simulink model "FCS_Design"  (R2024b)
settings: Solver=FixedStepDiscrete  StartTime=0.0  StopTime=10.0  RelTol=1e-3
settings OptimizationCC: DefaultParameterBehavior=Inlined  EnhancedBackFolding=on  PassReuseOutputArgsAs=Individual arguments  ZeroExternalMemoryAtStartup=off  ZeroInternalMemoryAtStartup=off  OptimizeBlockOrder=speed  DifferentSizesBufferReuse=on  OptimizationCustomize=off  EfficientTunableParamExpr=on
settings DebuggingCC: ParameterTunabilityLossMsg=error
settings SFSimCC: MATLABDynamicMemAlloc=off
settings RTWCC: Description=Embedded Coder  SystemTargetFile=ert.tlc  TemplateMakefile=ert_default_tmf
settings CodeAppCC: ForceParamTrailComments=on  IgnoreCustomStorageClasses=off  OperatorAnnotations=on  SimulinkDataObjDesc=on  SFDataObjDesc=on  InsertBlockDesc=on
settings ERTTargetCC: TargetLangStandard=C99 (ISO)  GenerateSampleERTMain=on  ERTCustomFileTemplate=example_file_process.tlc

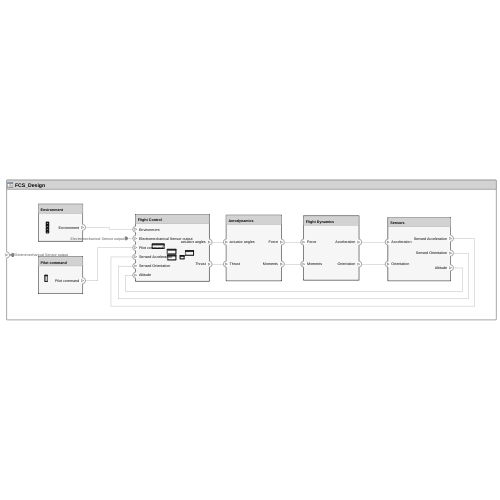
[thumbnail: Simulink's stored preview of the top-level diagram]
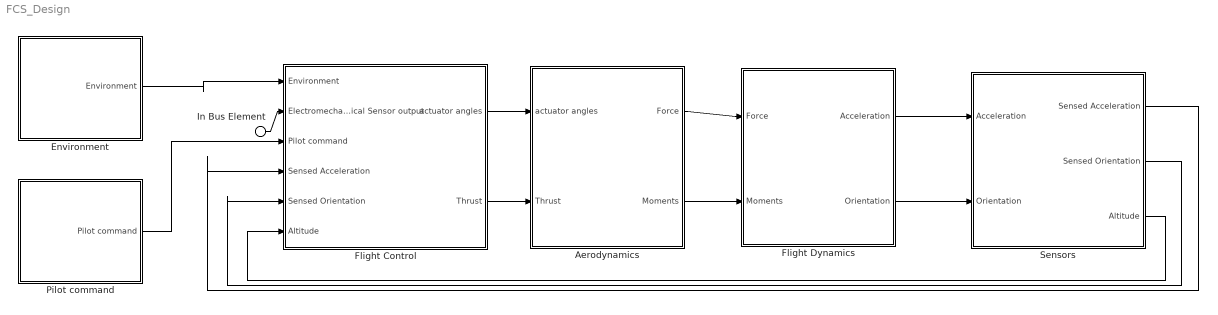
== system FCS_Design ==
  In Bus Element : Inport  PortName=Electromechanical Sensor output
  Aerodynamics : Subsystem
      settings: PortSchema="{\"entries\":[{\"content\":{\"headerSize\":26,\"margin\":15,\"minimumSpacing\":25,\"sides\":[{\"content\":{\"connectorIds\":[\"In1\",\"In2\"]},\"type\":\"ConnectorPlacement.EquallySpacedRectSide\",\"uuid\":\"d5d2077c-3b21-4d02-aba8-81a870ce330d\"},{\"content\":{\"connectorIds\":[\"Out1\",\"Out2\"],\"side\":\"RIGHT\"},\"type\":\"ConnectorPlacement.EquallySpacedRectSide\",\"uuid\":\"4fd2a41b-7df5-4294-829e-ab8ed7c0ae08\"},{\"content\":{\"side\":\"TOP\"},\"type\":\"ConnectorPlacement.EquallySpacedRectSide\",\"uuid\":\"02481d6b-9835-4bb6-a897-737025ba9b9d\"}]},\"type\":\"ConnectorPlacement.EquallySpacedConnector\",\"uuid\":\"7e1f026a-fb6c-4dac-9805-315e8c94a54c\"}],\"packageUris\":[\"http://schema.mathworks.com/mf0/Connector/R2020b\"],\"version\":\"1.0\"}"
  Environment : Subsystem
      settings: PortSchema="{\"entries\":[{\"content\":{\"headerSize\":26,\"margin\":15,\"minimumSpacing\":25,\"sides\":[{\"content\":{},\"type\":\"ConnectorPlacement.EquallySpacedRectSide\",\"uuid\":\"d5d2077c-3b21-4d02-aba8-81a870ce330d\"},{\"content\":{\"connectorIds\":[\"Out1\"],\"side\":\"RIGHT\"},\"type\":\"ConnectorPlacement.EquallySpacedRectSide\",\"uuid\":\"4fd2a41b-7df5-4294-829e-ab8ed7c0ae08\"},{\"content\":{\"side\":\"TOP\"},\"type\":\"ConnectorPlacement.EquallySpacedRectSide\",\"uuid\":\"02481d6b-9835-4bb6-a897-737025ba9b9d\"}]},\"type\":\"ConnectorPlacement.EquallySpacedConnector\",\"uuid\":\"7e1f026a-fb6c-4dac-9805-315e8c94a54c\"}],\"packageUris\":[\"http://schema.mathworks.com/mf0/Connector/R2020b\"],\"version\":\"1.0\"}"
  Flight Control : Subsystem
      settings: PortSchema="{\"entries\":[{\"content\":{\"headerSize\":26,\"margin\":15,\"minimumSpacing\":25,\"sides\":[{\"content\":{\"connectorIds\":[\"In1\",\"In2\",\"In3\",\"In4\",\"In5\",\"In6\"]},\"type\":\"ConnectorPlacement.EquallySpacedRectSide\",\"uuid\":\"d5d2077c-3b21-4d02-aba8-81a870ce330d\"},{\"content\":{\"connectorIds\":[\"Out1\",\"Out2\"],\"side\":\"RIGHT\"},\"type\":\"ConnectorPlacement.EquallySpacedRectSide\",\"uuid\":\"4fd2a41b-7df5-4294-829e-ab8ed7c0ae08\"},{\"content\":{\"side\":\"TOP\"},\"type\":\"ConnectorPlacement.EquallySpacedRectSide\",\"uuid\":\"02481d6b-9835-4bb6-a897-737025ba9b9d\"}]},\"type\":\"ConnectorPlacement.EquallySpacedConnector\",\"uuid\":\"7e1f026a-fb6c-4dac-9805-315e8c94a54c\"}],\"packageUris\":[\"http://schema.mathworks.com/mf0/Connector/R2020b\"],\"version\":\"1.0\"}"
  Flight Dynamics : Subsystem
      settings: PortSchema="{\"entries\":[{\"content\":{\"headerSize\":26,\"margin\":15,\"minimumSpacing\":25,\"sides\":[{\"content\":{\"connectorIds\":[\"In1\",\"In2\"]},\"type\":\"ConnectorPlacement.EquallySpacedRectSide\",\"uuid\":\"d5d2077c-3b21-4d02-aba8-81a870ce330d\"},{\"content\":{\"connectorIds\":[\"Out1\",\"Out2\"],\"side\":\"RIGHT\"},\"type\":\"ConnectorPlacement.EquallySpacedRectSide\",\"uuid\":\"4fd2a41b-7df5-4294-829e-ab8ed7c0ae08\"},{\"content\":{\"side\":\"TOP\"},\"type\":\"ConnectorPlacement.EquallySpacedRectSide\",\"uuid\":\"02481d6b-9835-4bb6-a897-737025ba9b9d\"}]},\"type\":\"ConnectorPlacement.EquallySpacedConnector\",\"uuid\":\"7e1f026a-fb6c-4dac-9805-315e8c94a54c\"}],\"packageUris\":[\"http://schema.mathworks.com/mf0/Connector/R2020b\"],\"version\":\"1.0\"}"
  Pilot command : Subsystem
      settings: PortSchema="{\"entries\":[{\"content\":{\"headerSize\":26,\"margin\":15,\"minimumSpacing\":25,\"sides\":[{\"content\":{},\"type\":\"ConnectorPlacement.EquallySpacedRectSide\",\"uuid\":\"d5d2077c-3b21-4d02-aba8-81a870ce330d\"},{\"content\":{\"connectorIds\":[\"Out1\"],\"side\":\"RIGHT\"},\"type\":\"ConnectorPlacement.EquallySpacedRectSide\",\"uuid\":\"4fd2a41b-7df5-4294-829e-ab8ed7c0ae08\"},{\"content\":{\"side\":\"TOP\"},\"type\":\"ConnectorPlacement.EquallySpacedRectSide\",\"uuid\":\"02481d6b-9835-4bb6-a897-737025ba9b9d\"}]},\"type\":\"ConnectorPlacement.EquallySpacedConnector\",\"uuid\":\"7e1f026a-fb6c-4dac-9805-315e8c94a54c\"}],\"packageUris\":[\"http://schema.mathworks.com/mf0/Connector/R2020b\"],\"version\":\"1.0\"}"
  Sensors : Subsystem
      settings: PortSchema="{\"entries\":[{\"content\":{\"headerSize\":26,\"margin\":15,\"minimumSpacing\":25,\"sides\":[{\"content\":{\"connectorIds\":[\"In1\",\"In2\"]},\"type\":\"ConnectorPlacement.EquallySpacedRectSide\",\"uuid\":\"d5d2077c-3b21-4d02-aba8-81a870ce330d\"},{\"content\":{\"connectorIds\":[\"Out1\",\"Out2\",\"Out3\"],\"side\":\"RIGHT\"},\"type\":\"ConnectorPlacement.EquallySpacedRectSide\",\"uuid\":\"4fd2a41b-7df5-4294-829e-ab8ed7c0ae08\"},{\"content\":{\"side\":\"TOP\"},\"type\":\"ConnectorPlacement.EquallySpacedRectSide\",\"uuid\":\"02481d6b-9835-4bb6-a897-737025ba9b9d\"}]},\"type\":\"ConnectorPlacement.EquallySpacedConnector\",\"uuid\":\"7e1f026a-fb6c-4dac-9805-315e8c94a54c\"}],\"packageUris\":[\"http://schema.mathworks.com/mf0/Connector/R2020b\"],\"version\":\"1.0\"}"
  wires:
  Flight Dynamics/1(Acceleration) -> Sensors/1(Acceleration)
  Flight Dynamics/2(Orientation) -> Sensors/2(Orientation)
  Sensors/3(Altitude) -> Flight Control/6(Altitude)
  Sensors/2(Sensed Orientation) -> Flight Control/5(Sensed Orientation)
  Sensors/1(Sensed Acceleration) -> Flight Control/4(Sensed Acceleration)
  Aerodynamics/1(Force) -> Flight Dynamics/1(Force)
  Aerodynamics/2(Moments) -> Flight Dynamics/2(Moments)
  Flight Control/1(actuator angles) -> Aerodynamics/1(actuator angles)
  Flight Control/2(Thrust) -> Aerodynamics/2(Thrust)
  Environment/1(Environment) -> Flight Control/1(Environment)
  Pilot command/1(Pilot command) -> Flight Control/3(Pilot command)
  In Bus Element/1 -> Flight Control/2(Electromechanical Sensor output)

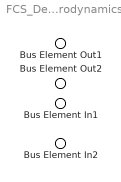
== system FCS_Design/Aerodynamics ==
  Bus Element In1 : Inport  PortName=actuator angles
  Bus Element In2 : Inport  Port=2  PortName=Thrust
  Bus Element Out1 : Outport  PortName=Force
  Bus Element Out2 : Outport  Port=2  PortName=Moments

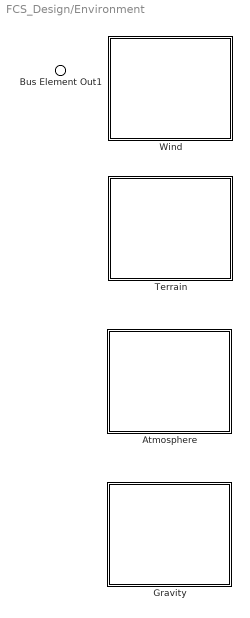
== system FCS_Design/Environment ==
  Atmosphere : Subsystem
      settings: PortSchema="{\"entries\":[{\"content\":{\"headerSize\":26,\"margin\":15,\"minimumSpacing\":25,\"sides\":[{\"content\":{},\"type\":\"ConnectorPlacement.EquallySpacedRectSide\",\"uuid\":\"d5d2077c-3b21-4d02-aba8-81a870ce330d\"},{\"content\":{\"side\":\"RIGHT\"},\"type\":\"ConnectorPlacement.EquallySpacedRectSide\",\"uuid\":\"4fd2a41b-7df5-4294-829e-ab8ed7c0ae08\"},{\"content\":{\"side\":\"TOP\"},\"type\":\"ConnectorPlacement.EquallySpacedRectSide\",\"uuid\":\"02481d6b-9835-4bb6-a897-737025ba9b9d\"}]},\"type\":\"ConnectorPlacement.EquallySpacedConnector\",\"uuid\":\"7e1f026a-fb6c-4dac-9805-315e8c94a54c\"}],\"packageUris\":[\"http://schema.mathworks.com/mf0/Connector/R2020b\"],\"version\":\"1.0\"}"
  Gravity : Subsystem
      settings: PortSchema="{\"entries\":[{\"content\":{\"headerSize\":26,\"margin\":15,\"minimumSpacing\":25,\"sides\":[{\"content\":{},\"type\":\"ConnectorPlacement.EquallySpacedRectSide\",\"uuid\":\"d5d2077c-3b21-4d02-aba8-81a870ce330d\"},{\"content\":{\"side\":\"RIGHT\"},\"type\":\"ConnectorPlacement.EquallySpacedRectSide\",\"uuid\":\"4fd2a41b-7df5-4294-829e-ab8ed7c0ae08\"},{\"content\":{\"side\":\"TOP\"},\"type\":\"ConnectorPlacement.EquallySpacedRectSide\",\"uuid\":\"02481d6b-9835-4bb6-a897-737025ba9b9d\"}]},\"type\":\"ConnectorPlacement.EquallySpacedConnector\",\"uuid\":\"7e1f026a-fb6c-4dac-9805-315e8c94a54c\"}],\"packageUris\":[\"http://schema.mathworks.com/mf0/Connector/R2020b\"],\"version\":\"1.0\"}"
  Terrain : Subsystem
      settings: PortSchema="{\"entries\":[{\"content\":{\"headerSize\":26,\"margin\":15,\"minimumSpacing\":25,\"sides\":[{\"content\":{},\"type\":\"ConnectorPlacement.EquallySpacedRectSide\",\"uuid\":\"d5d2077c-3b21-4d02-aba8-81a870ce330d\"},{\"content\":{\"side\":\"RIGHT\"},\"type\":\"ConnectorPlacement.EquallySpacedRectSide\",\"uuid\":\"4fd2a41b-7df5-4294-829e-ab8ed7c0ae08\"},{\"content\":{\"side\":\"TOP\"},\"type\":\"ConnectorPlacement.EquallySpacedRectSide\",\"uuid\":\"02481d6b-9835-4bb6-a897-737025ba9b9d\"}]},\"type\":\"ConnectorPlacement.EquallySpacedConnector\",\"uuid\":\"7e1f026a-fb6c-4dac-9805-315e8c94a54c\"}],\"packageUris\":[\"http://schema.mathworks.com/mf0/Connector/R2020b\"],\"version\":\"1.0\"}"
  Wind : Subsystem
      settings: PortSchema="{\"entries\":[{\"content\":{\"headerSize\":26,\"margin\":15,\"minimumSpacing\":25,\"sides\":[{\"content\":{},\"type\":\"ConnectorPlacement.EquallySpacedRectSide\",\"uuid\":\"d5d2077c-3b21-4d02-aba8-81a870ce330d\"},{\"content\":{\"side\":\"RIGHT\"},\"type\":\"ConnectorPlacement.EquallySpacedRectSide\",\"uuid\":\"4fd2a41b-7df5-4294-829e-ab8ed7c0ae08\"},{\"content\":{\"side\":\"TOP\"},\"type\":\"ConnectorPlacement.EquallySpacedRectSide\",\"uuid\":\"02481d6b-9835-4bb6-a897-737025ba9b9d\"}]},\"type\":\"ConnectorPlacement.EquallySpacedConnector\",\"uuid\":\"7e1f026a-fb6c-4dac-9805-315e8c94a54c\"}],\"packageUris\":[\"http://schema.mathworks.com/mf0/Connector/R2020b\"],\"version\":\"1.0\"}"
  Bus Element Out1 : Outport  PortName=Environment

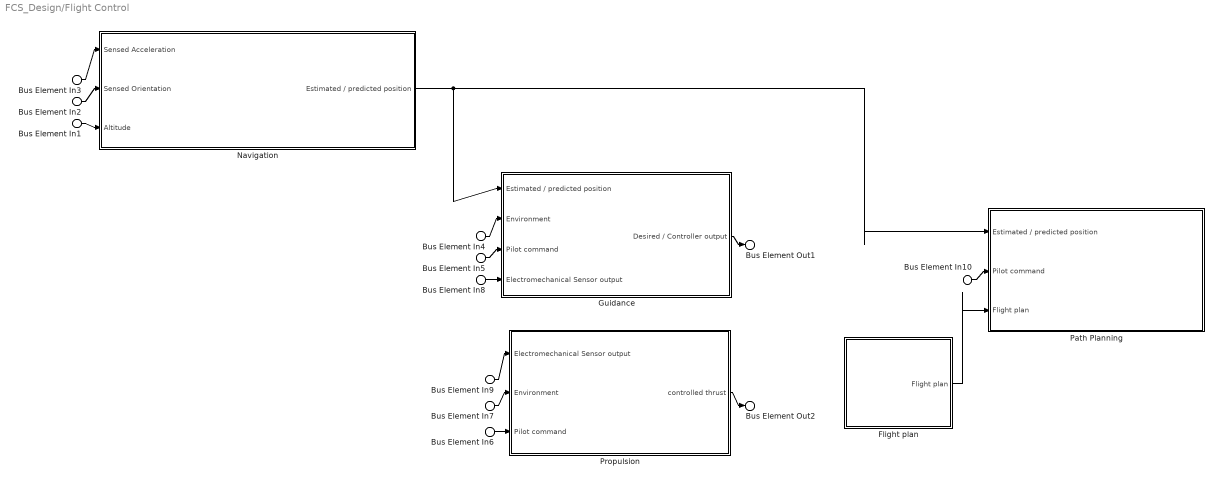
== system FCS_Design/Flight Control ==
  Bus Element In4 : Inport  PortName=Environment
  Bus Element In7 : Inport  PortName=Environment
  Bus Element In8 : Inport  Port=2  PortName=Electromechanical Sensor output
  Bus Element In9 : Inport  Port=2  PortName=Electromechanical Sensor output
  Bus Element In5 : Inport  Port=3  PortName=Pilot command
  Bus Element In6 : Inport  Port=3  PortName=Pilot command
  Bus Element In10 : Inport  Port=3  PortName=Pilot command
  Bus Element In3 : Inport  Port=4  PortName=Sensed Acceleration
  Bus Element In2 : Inport  Port=5  PortName=Sensed Orientation
  Bus Element In1 : Inport  Port=6  PortName=Altitude
  Flight plan : Subsystem
      settings: PortSchema="{\"entries\":[{\"content\":{\"headerSize\":26,\"margin\":15,\"minimumSpacing\":25,\"sides\":[{\"content\":{},\"type\":\"ConnectorPlacement.EquallySpacedRectSide\",\"uuid\":\"d5d2077c-3b21-4d02-aba8-81a870ce330d\"},{\"content\":{\"connectorIds\":[\"Out1\"],\"side\":\"RIGHT\"},\"type\":\"ConnectorPlacement.EquallySpacedRectSide\",\"uuid\":\"4fd2a41b-7df5-4294-829e-ab8ed7c0ae08\"},{\"content\":{\"side\":\"TOP\"},\"type\":\"ConnectorPlacement.EquallySpacedRectSide\",\"uuid\":\"02481d6b-9835-4bb6-a897-737025ba9b9d\"}]},\"type\":\"ConnectorPlacement.EquallySpacedConnector\",\"uuid\":\"7e1f026a-fb6c-4dac-9805-315e8c94a54c\"}],\"packageUris\":[\"http://schema.mathworks.com/mf0/Connector/R2020b\"],\"version\":\"1.0\"}"
  Guidance : Subsystem
      settings: PortSchema="{\"entries\":[{\"content\":{\"headerSize\":26,\"margin\":15,\"minimumSpacing\":25,\"sides\":[{\"content\":{\"connectorIds\":[\"In1\",\"In2\",\"In3\",\"In4\"]},\"type\":\"ConnectorPlacement.EquallySpacedRectSide\",\"uuid\":\"d5d2077c-3b21-4d02-aba8-81a870ce330d\"},{\"content\":{\"connectorIds\":[\"Out1\"],\"side\":\"RIGHT\"},\"type\":\"ConnectorPlacement.EquallySpacedRectSide\",\"uuid\":\"4fd2a41b-7df5-4294-829e-ab8ed7c0ae08\"},{\"content\":{\"side\":\"TOP\"},\"type\":\"ConnectorPlacement.EquallySpacedRectSide\",\"uuid\":\"02481d6b-9835-4bb6-a897-737025ba9b9d\"}]},\"type\":\"ConnectorPlacement.EquallySpacedConnector\",\"uuid\":\"7e1f026a-fb6c-4dac-9805-315e8c94a54c\"}],\"packageUris\":[\"http://schema.mathworks.com/mf0/Connector/R2020b\"],\"version\":\"1.0\"}"
  Navigation : Subsystem
      settings: PortSchema="{\"entries\":[{\"content\":{\"headerSize\":26,\"margin\":15,\"minimumSpacing\":25,\"sides\":[{\"content\":{\"connectorIds\":[\"In1\",\"In2\",\"In3\"]},\"type\":\"ConnectorPlacement.EquallySpacedRectSide\",\"uuid\":\"d5d2077c-3b21-4d02-aba8-81a870ce330d\"},{\"content\":{\"connectorIds\":[\"Out1\"],\"side\":\"RIGHT\"},\"type\":\"ConnectorPlacement.EquallySpacedRectSide\",\"uuid\":\"4fd2a41b-7df5-4294-829e-ab8ed7c0ae08\"},{\"content\":{\"side\":\"TOP\"},\"type\":\"ConnectorPlacement.EquallySpacedRectSide\",\"uuid\":\"02481d6b-9835-4bb6-a897-737025ba9b9d\"}]},\"type\":\"ConnectorPlacement.EquallySpacedConnector\",\"uuid\":\"7e1f026a-fb6c-4dac-9805-315e8c94a54c\"}],\"packageUris\":[\"http://schema.mathworks.com/mf0/Connector/R2020b\"],\"version\":\"1.0\"}"
  Path Planning : Subsystem
      settings: PortSchema="{\"entries\":[{\"content\":{\"headerSize\":26,\"margin\":15,\"minimumSpacing\":25,\"sides\":[{\"content\":{\"connectorIds\":[\"In1\",\"In2\",\"In3\"]},\"type\":\"ConnectorPlacement.EquallySpacedRectSide\",\"uuid\":\"d5d2077c-3b21-4d02-aba8-81a870ce330d\"},{\"content\":{\"side\":\"RIGHT\"},\"type\":\"ConnectorPlacement.EquallySpacedRectSide\",\"uuid\":\"4fd2a41b-7df5-4294-829e-ab8ed7c0ae08\"},{\"content\":{\"side\":\"TOP\"},\"type\":\"ConnectorPlacement.EquallySpacedRectSide\",\"uuid\":\"02481d6b-9835-4bb6-a897-737025ba9b9d\"}]},\"type\":\"ConnectorPlacement.EquallySpacedConnector\",\"uuid\":\"7e1f026a-fb6c-4dac-9805-315e8c94a54c\"}],\"packageUris\":[\"http://schema.mathworks.com/mf0/Connector/R2020b\"],\"version\":\"1.0\"}"
  "Propulsion " : Subsystem
      settings: PortSchema="{\"entries\":[{\"content\":{\"headerSize\":26,\"margin\":15,\"minimumSpacing\":25,\"sides\":[{\"content\":{\"connectorIds\":[\"In1\",\"In2\",\"In3\"]},\"type\":\"ConnectorPlacement.EquallySpacedRectSide\",\"uuid\":\"d5d2077c-3b21-4d02-aba8-81a870ce330d\"},{\"content\":{\"connectorIds\":[\"Out1\"],\"side\":\"RIGHT\"},\"type\":\"ConnectorPlacement.EquallySpacedRectSide\",\"uuid\":\"4fd2a41b-7df5-4294-829e-ab8ed7c0ae08\"},{\"content\":{\"side\":\"TOP\"},\"type\":\"ConnectorPlacement.EquallySpacedRectSide\",\"uuid\":\"02481d6b-9835-4bb6-a897-737025ba9b9d\"}]},\"type\":\"ConnectorPlacement.EquallySpacedConnector\",\"uuid\":\"7e1f026a-fb6c-4dac-9805-315e8c94a54c\"}],\"packageUris\":[\"http://schema.mathworks.com/mf0/Connector/R2020b\"],\"version\":\"1.0\"}"
  Bus Element Out1 : Outport  PortName=actuator angles
  Bus Element Out2 : Outport  Port=2  PortName=Thrust
  wires:
  Bus Element In3/1 -> Navigation/1(Sensed Acceleration)
  Bus Element In2/1 -> Navigation/2(Sensed Orientation)
  Bus Element In1/1 -> Navigation/3(Altitude)
  Bus Element In4/1 -> Guidance/2(Environment)
  Bus Element In5/1 -> Guidance/3(Pilot command)
  Bus Element In6/1 -> "Propulsion "/3(Pilot command)
  Bus Element In7/1 -> "Propulsion "/2(Environment)
  Bus Element In8/1 -> Guidance/4(Electromechanical Sensor output)
  Guidance/1(Desired / Controller output) -> Bus Element Out1/1
  Bus Element In9/1 -> "Propulsion "/1(Electromechanical Sensor output)
  "Propulsion "/1(controlled thrust) -> Bus Element Out2/1
  Bus Element In10/1 -> Path Planning/2(Pilot command)
  Navigation/1(Estimated / predicted position) -> Guidance/1(Estimated / predicted position), Path Planning/1(Estimated / predicted position)
  Flight plan/1(Flight plan) -> Path Planning/3(Flight plan)

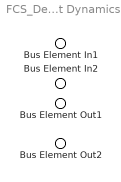
== system FCS_Design/Flight Dynamics ==
  Bus Element In1 : Inport  PortName=Force
  Bus Element In2 : Inport  Port=2  PortName=Moments
  Bus Element Out1 : Outport  PortName=Acceleration
  Bus Element Out2 : Outport  Port=2  PortName=Orientation

== system FCS_Design/Pilot command ==
  List fo Commands : Subsystem
      settings: PortSchema="{\"entries\":[{\"content\":{\"headerSize\":26,\"margin\":15,\"minimumSpacing\":25,\"sides\":[{\"content\":{},\"type\":\"ConnectorPlacement.EquallySpacedRectSide\",\"uuid\":\"d5d2077c-3b21-4d02-aba8-81a870ce330d\"},{\"content\":{\"connectorIds\":[\"Out1\",\"Out2\",\"Out3\",\"Out4\",\"Out5\",\"Out6\"],\"side\":\"RIGHT\"},\"type\":\"ConnectorPlacement.EquallySpacedRectSide\",\"uuid\":\"4fd2a41b-7df5-4294-829e-ab8ed7c0ae08\"},{\"content\":{\"side\":\"TOP\"},\"type\":\"ConnectorPlacement.EquallySpacedRectSide\",\"uuid\":\"02481d6b-9835-4bb6-a897-737025ba9b9d\"}]},\"type\":\"ConnectorPlacement.EquallySpacedConnector\",\"uuid\":\"7e1f026a-fb6c-4dac-9805-315e8c94a54c\"}],\"packageUris\":[\"http://schema.mathworks.com/mf0/Connector/R2020b\"],\"version\":\"1.0\"}"
  Bus Element Out1 : Outport  PortName=Pilot command

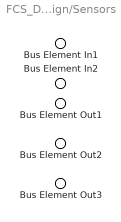
== system FCS_Design/Sensors ==
  Bus Element In1 : Inport  PortName=Acceleration
  Bus Element In2 : Inport  Port=2  PortName=Orientation
  Bus Element Out1 : Outport  PortName=Sensed Acceleration
  Bus Element Out2 : Outport  Port=2  PortName=Sensed Orientation
  Bus Element Out3 : Outport  Port=3  PortName=Altitude

== system FCS_Design/Environment/Atmosphere ==

== system FCS_Design/Environment/Gravity ==

== system FCS_Design/Environment/Terrain ==

== system FCS_Design/Environment/Wind ==

== system FCS_Design/Flight Control/Flight plan ==
  Bus Element Out1 : Outport  PortName=Flight plan

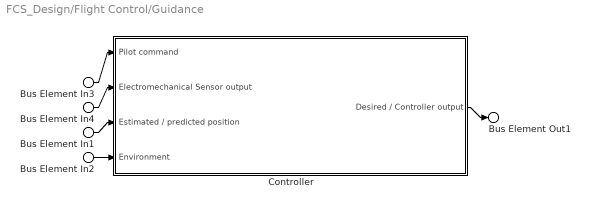
== system FCS_Design/Flight Control/Guidance ==
  Bus Element In1 : Inport  PortName=Estimated / predicted position
  Bus Element In2 : Inport  Port=2  PortName=Environment
  Bus Element In3 : Inport  Port=3  PortName=Pilot command
  Bus Element In4 : Inport  Port=4  PortName=Electromechanical Sensor output
  Controller : Subsystem
      settings: PortSchema="{\"entries\":[{\"content\":{\"headerSize\":26,\"margin\":15,\"minimumSpacing\":25,\"sides\":[{\"content\":{\"connectorIds\":[\"In1\",\"In2\",\"In3\",\"In4\"]},\"type\":\"ConnectorPlacement.EquallySpacedRectSide\",\"uuid\":\"d5d2077c-3b21-4d02-aba8-81a870ce330d\"},{\"content\":{\"connectorIds\":[\"Out1\"],\"side\":\"RIGHT\"},\"type\":\"ConnectorPlacement.EquallySpacedRectSide\",\"uuid\":\"4fd2a41b-7df5-4294-829e-ab8ed7c0ae08\"},{\"content\":{\"side\":\"TOP\"},\"type\":\"ConnectorPlacement.EquallySpacedRectSide\",\"uuid\":\"02481d6b-9835-4bb6-a897-737025ba9b9d\"}]},\"type\":\"ConnectorPlacement.EquallySpacedConnector\",\"uuid\":\"7e1f026a-fb6c-4dac-9805-315e8c94a54c\"}],\"packageUris\":[\"http://schema.mathworks.com/mf0/Connector/R2020b\"],\"version\":\"1.0\"}"
  Bus Element Out1 : Outport  PortName=Desired / Controller output
  wires:
  Bus Element In3/1 -> Controller/1(Pilot command)
  Bus Element In4/1 -> Controller/2(Electromechanical Sensor output)
  Bus Element In1/1 -> Controller/3(Estimated / predicted position)
  Bus Element In2/1 -> Controller/4(Environment)
  Controller/1(Desired / Controller output) -> Bus Element Out1/1

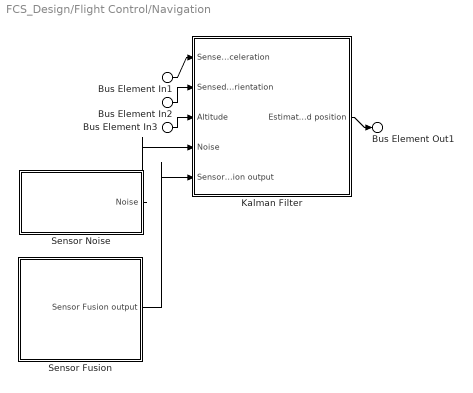
== system FCS_Design/Flight Control/Navigation ==
  Bus Element In1 : Inport  PortName=Sensed Acceleration
  Bus Element In2 : Inport  Port=2  PortName=Sensed Orientation
  Bus Element In3 : Inport  Port=3  PortName=Altitude
  Kalman Filter : Subsystem
      settings: PortSchema="{\"entries\":[{\"content\":{\"headerSize\":26,\"margin\":15,\"minimumSpacing\":25,\"sides\":[{\"content\":{\"connectorIds\":[\"In1\",\"In2\",\"In3\",\"In4\",\"In5\"]},\"type\":\"ConnectorPlacement.EquallySpacedRectSide\",\"uuid\":\"d5d2077c-3b21-4d02-aba8-81a870ce330d\"},{\"content\":{\"connectorIds\":[\"Out1\"],\"side\":\"RIGHT\"},\"type\":\"ConnectorPlacement.EquallySpacedRectSide\",\"uuid\":\"4fd2a41b-7df5-4294-829e-ab8ed7c0ae08\"},{\"content\":{\"side\":\"TOP\"},\"type\":\"ConnectorPlacement.EquallySpacedRectSide\",\"uuid\":\"02481d6b-9835-4bb6-a897-737025ba9b9d\"}]},\"type\":\"ConnectorPlacement.EquallySpacedConnector\",\"uuid\":\"7e1f026a-fb6c-4dac-9805-315e8c94a54c\"}],\"packageUris\":[\"http://schema.mathworks.com/mf0/Connector/R2020b\"],\"version\":\"1.0\"}"
  Sensor Fusion : Subsystem
      settings: PortSchema="{\"entries\":[{\"content\":{\"headerSize\":26,\"margin\":15,\"minimumSpacing\":25,\"sides\":[{\"content\":{},\"type\":\"ConnectorPlacement.EquallySpacedRectSide\",\"uuid\":\"d5d2077c-3b21-4d02-aba8-81a870ce330d\"},{\"content\":{\"connectorIds\":[\"Out1\"],\"side\":\"RIGHT\"},\"type\":\"ConnectorPlacement.EquallySpacedRectSide\",\"uuid\":\"4fd2a41b-7df5-4294-829e-ab8ed7c0ae08\"},{\"content\":{\"side\":\"TOP\"},\"type\":\"ConnectorPlacement.EquallySpacedRectSide\",\"uuid\":\"02481d6b-9835-4bb6-a897-737025ba9b9d\"}]},\"type\":\"ConnectorPlacement.EquallySpacedConnector\",\"uuid\":\"7e1f026a-fb6c-4dac-9805-315e8c94a54c\"}],\"packageUris\":[\"http://schema.mathworks.com/mf0/Connector/R2020b\"],\"version\":\"1.0\"}"
  Sensor Noise : Subsystem
      settings: PortSchema="{\"entries\":[{\"content\":{\"headerSize\":26,\"margin\":15,\"minimumSpacing\":25,\"sides\":[{\"content\":{},\"type\":\"ConnectorPlacement.EquallySpacedRectSide\",\"uuid\":\"d5d2077c-3b21-4d02-aba8-81a870ce330d\"},{\"content\":{\"connectorIds\":[\"Out1\"],\"side\":\"RIGHT\"},\"type\":\"ConnectorPlacement.EquallySpacedRectSide\",\"uuid\":\"4fd2a41b-7df5-4294-829e-ab8ed7c0ae08\"},{\"content\":{\"side\":\"TOP\"},\"type\":\"ConnectorPlacement.EquallySpacedRectSide\",\"uuid\":\"02481d6b-9835-4bb6-a897-737025ba9b9d\"}]},\"type\":\"ConnectorPlacement.EquallySpacedConnector\",\"uuid\":\"7e1f026a-fb6c-4dac-9805-315e8c94a54c\"}],\"packageUris\":[\"http://schema.mathworks.com/mf0/Connector/R2020b\"],\"version\":\"1.0\"}"
  Bus Element Out1 : Outport  PortName=Estimated / predicted position
  wires:
  Bus Element In1/1 -> Kalman Filter/1(Sensed Acceleration)
  Bus Element In2/1 -> Kalman Filter/2(Sensed Orientation)
  Bus Element In3/1 -> Kalman Filter/3(Altitude)
  Sensor Noise/1(Noise) -> Kalman Filter/4(Noise)
  Sensor Fusion/1(Sensor Fusion output) -> Kalman Filter/5(Sensor Fusion output)
  Kalman Filter/1(Estimated position) -> Bus Element Out1/1

== system FCS_Design/Flight Control/Path Planning ==
  Bus Element In2 : Inport  PortName=Estimated / predicted position
  Bus Element In1 : Inport  Port=2  PortName=Pilot command
  Bus Element In3 : Inport  Port=3  PortName=Flight plan

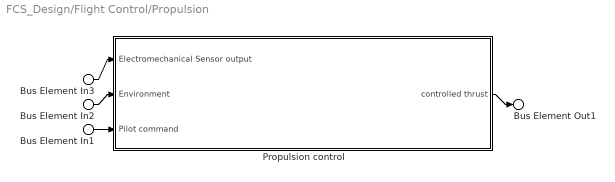
== system FCS_Design/Flight Control/Propulsion  ==
  Bus Element In3 : Inport  PortName=Electromechanical Sensor output
  Bus Element In2 : Inport  Port=2  PortName=Environment
  Bus Element In1 : Inport  Port=3  PortName=Pilot command
  Propulsion control : Subsystem
      settings: PortSchema="{\"entries\":[{\"content\":{\"headerSize\":26,\"margin\":15,\"minimumSpacing\":25,\"sides\":[{\"content\":{\"connectorIds\":[\"In1\",\"In2\",\"In3\"]},\"type\":\"ConnectorPlacement.EquallySpacedRectSide\",\"uuid\":\"d5d2077c-3b21-4d02-aba8-81a870ce330d\"},{\"content\":{\"connectorIds\":[\"Out1\"],\"side\":\"RIGHT\"},\"type\":\"ConnectorPlacement.EquallySpacedRectSide\",\"uuid\":\"4fd2a41b-7df5-4294-829e-ab8ed7c0ae08\"},{\"content\":{\"side\":\"TOP\"},\"type\":\"ConnectorPlacement.EquallySpacedRectSide\",\"uuid\":\"02481d6b-9835-4bb6-a897-737025ba9b9d\"}]},\"type\":\"ConnectorPlacement.EquallySpacedConnector\",\"uuid\":\"7e1f026a-fb6c-4dac-9805-315e8c94a54c\"}],\"packageUris\":[\"http://schema.mathworks.com/mf0/Connector/R2020b\"],\"version\":\"1.0\"}"
  Bus Element Out1 : Outport  PortName=controlled thrust
  wires:
  Bus Element In3/1 -> Propulsion control/1(Electromechanical Sensor output)
  Bus Element In2/1 -> Propulsion control/2(Environment)
  Bus Element In1/1 -> Propulsion control/3(Pilot command)
  Propulsion control/1(controlled thrust) -> Bus Element Out1/1

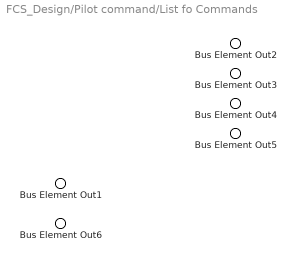
== system FCS_Design/Pilot command/List fo Commands ==
  Bus Element Out2 : Outport  PortName=Aileron
  Bus Element Out4 : Outport  Port=2  PortName=Elevator
  Bus Element Out3 : Outport  Port=3  PortName=Rudder
  Bus Element Out5 : Outport  Port=4  PortName=Heading
  Bus Element Out1 : Outport  Port=5  PortName=Throttle
  Bus Element Out6 : Outport  Port=6  PortName=Altitude

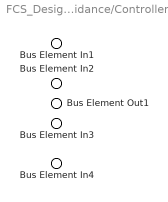
== system FCS_Design/Flight Control/Guidance/Controller ==
  Bus Element In1 : Inport  PortName=Pilot command
  Bus Element In2 : Inport  Port=2  PortName=Electromechanical Sensor output
  Bus Element In3 : Inport  Port=3  PortName=Estimated / predicted position
  Bus Element In4 : Inport  Port=4  PortName=Environment
  Bus Element Out1 : Outport  PortName=Desired / Controller output

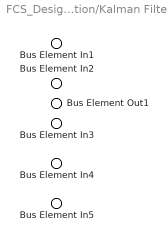
== system FCS_Design/Flight Control/Navigation/Kalman Filter ==
  Bus Element In1 : Inport  PortName=Sensed Acceleration
  Bus Element In2 : Inport  Port=2  PortName=Sensed Orientation
  Bus Element In3 : Inport  Port=3  PortName=Altitude
  Bus Element In4 : Inport  Port=4  PortName=Noise
  Bus Element In5 : Inport  Port=5  PortName=Sensor Fusion output
  Bus Element Out1 : Outport  PortName=Estimated position

== system FCS_Design/Flight Control/Navigation/Sensor Fusion ==
  Bus Element Out1 : Outport  PortName=Sensor Fusion output

== system FCS_Design/Flight Control/Navigation/Sensor Noise ==
  Bus Element Out1 : Outport  PortName=Noise

== system FCS_Design/Flight Control/Propulsion /Propulsion control ==
  Bus Element In1 : Inport  PortName=Electromechanical Sensor output
  Bus Element In2 : Inport  Port=2  PortName=Environment
  Bus Element In3 : Inport  Port=3  PortName=Pilot command
  Bus Element Out1 : Outport  PortName=controlled thrust
